simulink model "pich_pid"  (Simulink 7.7)
settings: Solver=ode3  StartTime=0.0  StopTime=100  FixedStep=0.1  RelTol=1e-6
PreLoadFcn:
  | load tras_char
values from neighbouring files (symbols this model uses):
  control_p = [-1,-0.975000000000000,-0.950000000000000,-0.925000000000000,-0.900000000000000,-0.875000000000000,-0.850000000000000,-0.825000000000000,-0.800000000000000,-0.775000000000000,-0.750000000000000,-0.725000000000000,-0.700000000000000,-0.675000000000000,-0.650000000000000,-0.625000000000000,-0.600000000000000,-0.575000000000000,-0.550000000000000,-0.525000000000000,-0.500000000000000,-0.4750000000000 ...(+1058 chars)    [main.m]
  force_p = [-0.714170782059585,-0.698541481136658,-0.676359428972366,-0.657306593399180,-0.636149510200777,-0.615949677515112,-0.602138570676813,-0.585879142379102,-0.565408182885363,-0.543655801354706,-0.527755120628238,-0.502405059234672,-0.485276085519214,-0.468134124703152,-0.445933772533463,-0.427151136118307,-0.408462867012090,-0.386931266191710,-0.367853637062824,-0.349068470693005,-0.324248856460492, ...(+1121 chars)    [main.m]
  GCE = GE*(Kp-sqrt(Kp^2-4*Ki*Kd))/2/Ki    [main.m]
  GCU = Ki/GE    (= 0.001)    [main.m]
  GE = 1    [main.m]
  GU = Kd/GCE    [main.m]
  rpm_p = [-3941.33990805745,-3812.34781047405,-3751.11151919774,-3716.53325007516,-3652.15015900441,-3605.21060614596,-3541.61821912219,-3501.87845652477,-3434.16395565290,-3361.65746230900,-3323.64747018525,-3262.37352633531,-3200.40694372361,-3113.97714681560,-3066.79116629220,-2985.72573717380,-2938.26747796475,-2854.00073711688,-2797.89727840112,-2739.44446768238,-2641.03778047718,-2564.22034843818,-24 ...(+1020 chars)    [main.m]
  Ts = 0.1    [main.m]
undefined symbols (not defined in the file or in its folder): DiscIntNeverNeededParam
libraries: simulink x2, fuzblock x1
settings Model: Creator=melanholly  LastModifiedBy=melanholly
settings DataIOCC: SignalLoggingName=sigsOut
settings DebuggingCC: SaveWithParameterizedLinksMsg=none  SignalResolutionControl=TryResolveAllWithWarning  SolverPrmCheckMsg=none  MultiTaskDSMMsg=warning  MultiTaskCondExecSysMsg=none  StrictBusMsg=None
settings HardwareCC: TargetUnknown=on
settings RTWCC: IncludeERTFirstTime=on

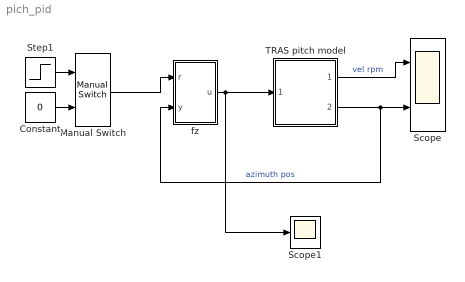
== system pich_pid ==
  Constant : Constant  Value=0
  Manual Switch : simulink/Signal Routing/Manual Switch  SystemSampleTime=-1  sw=1  action=0  varsize=off
  Scope : Scope  NumInputPorts=2
      settings: YMin=-5~-5  YMax=5~5
  Scope1 : Scope
      settings: TimeRange=12  YMin=0  YMax=1.223758865248227
  Step1 : Step  Time=50  Before=0.3  After=0.5  SampleTime=0
  TRAS pitch model : Subsystem
  fz : Subsystem
  wires:
  TRAS pitch model/1(rpm_p) -> Scope/1  "vel rpm"
  TRAS pitch model/2(pos_pm) -> Scope/2, fz/2(y)  "azimuth pos"
  Manual Switch/1 -> fz/1(r)
  Step1/1 -> Manual Switch/1
  Constant/1 -> Manual Switch/2
  fz/1(u) -> Scope1/1, TRAS pitch model/1(ctrl_p)

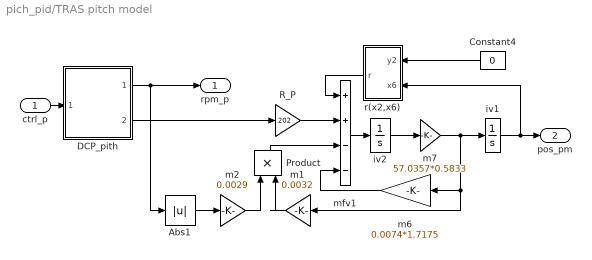
== system pich_pid/TRAS pitch model ==
  ctrl_p : Inport
  Abs1 : Abs  SaturateOnIntegerOverflow=on
  Constant4 : Constant  Value=0
  DCP_pith : Subsystem
  Product : Product  SaturateOnIntegerOverflow=on  OutDataTypeStr=Inherit: Same as first input
  R_P : Gain  Gain=.202  OutDataTypeStr=Inherit: Same as input  ParamDataTypeStr=Inherit: Same as input
  iv1 : Integrator  LimitOutput=on  UpperSaturationLimit=pi/2  LowerSaturationLimit=-pi/2
  iv2 : Integrator  InitialCondition=-.1  UpperSaturationLimit=pi  LowerSaturationLimit=-pi
  m1 : Gain  Gain=0.0032  SaturateOnIntegerOverflow=on  OutDataTypeStr=Inherit: Same as input  ParamDataTypeStr=Inherit: Same as input
  m2 : Gain  Gain=0.0029  SaturateOnIntegerOverflow=on  OutDataTypeStr=Inherit: Same as input  ParamDataTypeStr=Inherit: Same as input
  m6 : Gain  Gain=0.0074*1.7175  OutDataTypeStr=Inherit: Same as input  ParamDataTypeStr=Inherit: Same as input
  m7 : Gain  Gain=57.0357*0.5833  SaturateOnIntegerOverflow=on  OutDataTypeStr=Inherit: Same as input  ParamDataTypeStr=Inherit: Same as input
  mfv1 : Sum  Inputs=++--  SaturateOnIntegerOverflow=on  InputSameDT=on  OutDataTypeStr=Inherit: Same as first input
  r(x2,x6) : Subsystem
  rpm_p : Outport
  pos_pm : Outport  Port=2
  wires:
  ctrl_p/1 -> DCP_pith/1(CTR_P)
  mfv1/1 -> iv2/1
  m2/1 -> Product/1
  m1/1 -> Product/2
  Constant4/1 -> r(x2,x6)/1(y2)
  r(x2,x6)/1(r) -> mfv1/1
  Product/1 -> mfv1/3
  Abs1/1 -> m2/1
  DCP_pith/1(RPM_P) -> rpm_p/1, Abs1/1
  m7/1 -> iv1/1, m6/1, m1/1
  iv2/1 -> m7/1
  m6/1 -> mfv1/4
  DCP_pith/2(FORCE_P) -> R_P/1
  R_P/1 -> mfv1/2
  iv1/1 -> pos_pm/1, r(x2,x6)/2(x6)

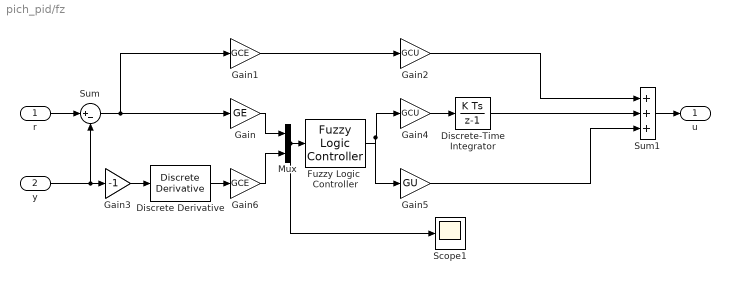
== system pich_pid/fz ==
  r : Inport
  y : Inport  Port=2
  Discrete Derivative : simulink/Discrete/Discrete Derivative  SystemSampleTime=-1  gainval=1.0  ICPrevScaledInput=0.0  OutMin=[]  OutMax=[]  OutDataType=fixdt(1, 16)  OutScaling=2^-10  DoSatur=off
  Discrete-Time Integrator : DiscreteIntegrator  SampleTime=Ts  ICPrevOutput=DiscIntNeverNeededParam  ICPrevScaledInput=DiscIntNeverNeededParam
  Fuzzy Logic  Controller : fuzblock/Fuzzy Logic  Controller  SystemSampleTime=-1  fis=FIS
  Gain : Gain  Gain=GE  SampleTime=Ts
  Gain1 : Gain  Gain=GCE  SampleTime=Ts
  Gain2 : Gain  Gain=GCU  SampleTime=Ts
  Gain3 : Gain  Gain=-1  SampleTime=Ts
  Gain4 : Gain  Gain=GCU  SampleTime=Ts
  Gain5 : Gain  Gain=GU  SampleTime=Ts
  Gain6 : Gain  Gain=GCE  SampleTime=Ts
  Mux : Mux  Inputs=2
  Scope1 : Scope
      settings: TimeRange=12  YMin=0  YMax=1.223758865248227  SaveName=ScopeData2
  Sum : Sum  Inputs=|+-
  Sum1 : Sum  Inputs=+++
  u : Outport
  wires:
  Gain6/1 -> Mux/2
  Gain/1 -> Mux/1
  Mux/1 -> Fuzzy Logic  Controller/1, Scope1/1
  Discrete Derivative/1 -> Gain6/1
  Gain5/1 -> Sum1/3
  Gain4/1 -> Discrete-Time Integrator/1
  Gain2/1 -> Sum1/1
  Gain1/1 -> Gain2/1
  y/1 -> Sum/2, Gain3/1
  Sum/1 -> Gain1/1, Gain/1
  Discrete-Time Integrator/1 -> Sum1/2
  Fuzzy Logic  Controller/1 -> Gain4/1, Gain5/1
  Gain3/1 -> Discrete Derivative/1
  r/1 -> Sum/1
  Sum1/1 -> u/1

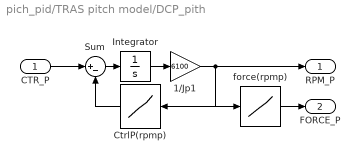
== system pich_pid/TRAS pitch model/DCP_pith ==
  CTR_P : Inport
  1/Jp1 : Gain  Gain=6100  OutDataTypeStr=Inherit: Same as input  ParamDataTypeStr=Inherit: Same as input
  CtrlP(rpmp) : Lookup  InputValues=rpm_p  Table=control_p  SaturateOnIntegerOverflow=on
  Integrator : Integrator
  Sum : Sum  Inputs=|+-  SampleTime=Ts  SaturateOnIntegerOverflow=on  InputSameDT=on  OutDataTypeStr=Inherit: Same as first input
  force(rpmp) : Lookup  InputValues=rpm_p  Table=force_p  SaturateOnIntegerOverflow=on
  RPM_P : Outport
  FORCE_P : Outport  Port=2
  wires:
  force(rpmp)/1 -> FORCE_P/1
  CTR_P/1 -> Sum/1
  1/Jp1/1 -> RPM_P/1, force(rpmp)/1, CtrlP(rpmp)/1
  CtrlP(rpmp)/1 -> Sum/2
  Integrator/1 -> 1/Jp1/1
  Sum/1 -> Integrator/1

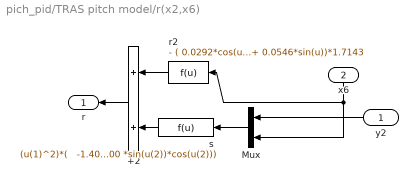
== system pich_pid/TRAS pitch model/r(x2,x6) ==
  y2 : Inport
  x6 : Inport  Port=2
  +2 : Sum  SaturateOnIntegerOverflow=on  InputSameDT=on  OutDataTypeStr=Inherit: Same as first input
  Mux : Mux  Inputs=2
  r2 : Fcn  Expr=- ( 0.0292*cos(u)+ 0.0546*sin(u))*1.7143
  s : Fcn  Expr="(u(1)^2)*(   -1.40920355960000 *sin(u(2))*cos(u(2)))"
  r : Outport
  wires:
  +2/1 -> r/1
  y2/1 -> Mux/1
  x6/1 -> r2/1, Mux/2
  s/1 -> +2/2
  r2/1 -> +2/1
  Mux/1 -> s/1
